simulink model "SF021A_HwAgTrajGenn"  (R2013b)
settings: Solver=FixedStepDiscrete  SolverMode=SingleTasking  StartTime=0.0  StopTime=1  FixedStep=0.002  RelTol=1e-3
undefined symbols (not defined in the file): ARCHGLBPRM_2MILLISEC_SEC_F32, HwAgTrajCmdSt1, HwAgTrajGennAgMax, HwAgTrajGennAMax, HwAgTrajGennVelMax, MINATAR_HWDEGPERSECPERSEC_F32, MINVELTAR_HWDEGPERSEC_F32, SYSGLBPRM_HWAGHILIM_HWDEG_F32, SYSGLBPRM_HWAGLOLIM_HWDEG_F32
libraries: simulink x13, NexteerUtilities x5
(part 2 of 2)

== system SF021A_HwAgTrajGenn/HwAgTrajGenn/HwAgTrajGennPer1/Generate Signals/Case 1/If Action Subsystem1 ==
  Cmd_St : Inport
  Ti_St : Inport  Port=2
  HwPosn_Offs : Inport  Port=3
  Action Port : ActionPort  ActionType=else
  CopyRight2 : Subsystem  Description=|  mask(Copyright Information){none=on}
      | Copyright info block.                                               
      |                                                                     
      | Place copyright information at the top of every subsystem in design.
      mask prompts: none "No parameters"
      mask help: Place copyright information at the top of every subsystem in design.
      mask Display:
      | NxtrConf = 'Nexteer Confidential';
      | 
      | sys = bdroot; %handle for the current model ("system")
      | first = get_param(sys,'Created');
      | if(isempty(first))
      |     first = datestr(now,'yyyy');
      | else
      |     first = first(end-3:end);  %year is last four digits
      | end
      | 
      | last = get_param(sys,'LastModifiedDate');
      | if isempty(last)
      |     last = datestr(now,'yyyy');
      | else
      |     last = last(end-3:end);
      | end
      | 
      | if strcmp(first,last)
      |     fprintf('%s -- Copyright %s Nexteer',NxtrConf,first)
      | else
      |     fprintf('%s -- %s%s- %s Nexteer',NxtrConf,char(169),first,last)
      | end
  Cmd_St_notDone : Outport
  Ti_St_notDone : Outport  Port=2
  HwPosn_Offs_notDone : Outport  Port=3
  wires:
  HwPosn_Offs/1 -> HwPosn_Offs_notDone/1
  Ti_St/1 -> Ti_St_notDone/1
  Cmd_St/1 -> Cmd_St_notDone/1

== system SF021A_HwAgTrajGenn/HwAgTrajGenn/HwAgTrajGennPer1/Generate Signals/Case 2/CopyRight2 ==

== system SF021A_HwAgTrajGenn/HwAgTrajGenn/HwAgTrajGennPer1/Generate Signals/Case 2/If Action Subsystem ==
  Cmd_St : Inport
  Ti_St : Inport  Port=2
  HwPosn_Offs : Inport  Port=3
  Action Port : ActionPort  ActionType=then
  CopyRight2 : Subsystem  Description=|  mask(Copyright Information){none=on}
      | Copyright info block.                                               
      |                                                                     
      | Place copyright information at the top of every subsystem in design.
      mask prompts: none "No parameters"
      mask help: Place copyright information at the top of every subsystem in design.
      mask Display:
      | NxtrConf = 'Nexteer Confidential';
      | 
      | sys = bdroot; %handle for the current model ("system")
      | first = get_param(sys,'Created');
      | if(isempty(first))
      |     first = datestr(now,'yyyy');
      | else
      |     first = first(end-3:end);  %year is last four digits
      | end
      | 
      | last = get_param(sys,'LastModifiedDate');
      | if isempty(last)
      |     last = datestr(now,'yyyy');
      | else
      |     last = last(end-3:end);
      | end
      | 
      | if strcmp(first,last)
      |     fprintf('%s -- Copyright %s Nexteer',NxtrConf,first)
      | else
      |     fprintf('%s -- %s%s- %s Nexteer',NxtrConf,char(169),first,last)
      | end
  Cmd_St_Done : Outport
  Ti_St_Done : Outport  Port=2
  HwPosn_Offs_Done : Outport  Port=3
  wires:
  HwPosn_Offs/1 -> HwPosn_Offs_Done/1
  Ti_St/1 -> Ti_St_Done/1
  Cmd_St/1 -> Cmd_St_Done/1

== system SF021A_HwAgTrajGenn/HwAgTrajGenn/HwAgTrajGennPer1/Generate Signals/Case 2/If Action Subsystem1 ==
  Cmd_St : Inport
  Ti_St : Inport  Port=2
  HwPosn_Offs : Inport  Port=3
  Action Port : ActionPort  ActionType=else
  CopyRight2 : Subsystem  Description=|  mask(Copyright Information){none=on}
      | Copyright info block.                                               
      |                                                                     
      | Place copyright information at the top of every subsystem in design.
      mask prompts: none "No parameters"
      mask help: Place copyright information at the top of every subsystem in design.
      mask Display:
      | NxtrConf = 'Nexteer Confidential';
      | 
      | sys = bdroot; %handle for the current model ("system")
      | first = get_param(sys,'Created');
      | if(isempty(first))
      |     first = datestr(now,'yyyy');
      | else
      |     first = first(end-3:end);  %year is last four digits
      | end
      | 
      | last = get_param(sys,'LastModifiedDate');
      | if isempty(last)
      |     last = datestr(now,'yyyy');
      | else
      |     last = last(end-3:end);
      | end
      | 
      | if strcmp(first,last)
      |     fprintf('%s -- Copyright %s Nexteer',NxtrConf,first)
      | else
      |     fprintf('%s -- %s%s- %s Nexteer',NxtrConf,char(169),first,last)
      | end
  Cmd_St_notDone : Outport
  Ti_St_notDone : Outport  Port=2
  HwPosn_Offs_notDone : Outport  Port=3
  wires:
  Cmd_St/1 -> Cmd_St_notDone/1
  Ti_St/1 -> Ti_St_notDone/1
  HwPosn_Offs/1 -> HwPosn_Offs_notDone/1

== system SF021A_HwAgTrajGenn/HwAgTrajGenn/HwAgTrajGennPer1/Generate Signals/Case 3/CopyRight2 ==

== system SF021A_HwAgTrajGenn/HwAgTrajGenn/HwAgTrajGennPer1/Generate Signals/Case 3/If Action Subsystem ==
  Cmd_St : Inport
  Ti_St : Inport  Port=2
  HwPosn_Offs : Inport  Port=3
  Action Port : ActionPort  ActionType=then
  CopyRight2 : Subsystem  Description=|  mask(Copyright Information){none=on}
      | Copyright info block.                                               
      |                                                                     
      | Place copyright information at the top of every subsystem in design.
      mask prompts: none "No parameters"
      mask help: Place copyright information at the top of every subsystem in design.
      mask Display:
      | NxtrConf = 'Nexteer Confidential';
      | 
      | sys = bdroot; %handle for the current model ("system")
      | first = get_param(sys,'Created');
      | if(isempty(first))
      |     first = datestr(now,'yyyy');
      | else
      |     first = first(end-3:end);  %year is last four digits
      | end
      | 
      | last = get_param(sys,'LastModifiedDate');
      | if isempty(last)
      |     last = datestr(now,'yyyy');
      | else
      |     last = last(end-3:end);
      | end
      | 
      | if strcmp(first,last)
      |     fprintf('%s -- Copyright %s Nexteer',NxtrConf,first)
      | else
      |     fprintf('%s -- %s%s- %s Nexteer',NxtrConf,char(169),first,last)
      | end
  Cmd_St_Done : Outport
  Ti_St_Done : Outport  Port=2
  HwPosn_Offs_Done : Outport  Port=3
  wires:
  HwPosn_Offs/1 -> HwPosn_Offs_Done/1
  Ti_St/1 -> Ti_St_Done/1
  Cmd_St/1 -> Cmd_St_Done/1

== system SF021A_HwAgTrajGenn/HwAgTrajGenn/HwAgTrajGennPer1/Generate Signals/Case 3/If Action Subsystem1 ==
  Cmd_St : Inport
  Ti_St : Inport  Port=2
  HwPosn_Offs : Inport  Port=3
  Action Port : ActionPort  ActionType=else
  CopyRight2 : Subsystem  Description=|  mask(Copyright Information){none=on}
      | Copyright info block.                                               
      |                                                                     
      | Place copyright information at the top of every subsystem in design.
      mask prompts: none "No parameters"
      mask help: Place copyright information at the top of every subsystem in design.
      mask Display:
      | NxtrConf = 'Nexteer Confidential';
      | 
      | sys = bdroot; %handle for the current model ("system")
      | first = get_param(sys,'Created');
      | if(isempty(first))
      |     first = datestr(now,'yyyy');
      | else
      |     first = first(end-3:end);  %year is last four digits
      | end
      | 
      | last = get_param(sys,'LastModifiedDate');
      | if isempty(last)
      |     last = datestr(now,'yyyy');
      | else
      |     last = last(end-3:end);
      | end
      | 
      | if strcmp(first,last)
      |     fprintf('%s -- Copyright %s Nexteer',NxtrConf,first)
      | else
      |     fprintf('%s -- %s%s- %s Nexteer',NxtrConf,char(169),first,last)
      | end
  Cmd_St_notDone : Outport
  Ti_St_notDone : Outport  Port=2
  HwPosn_Offs_notDone : Outport  Port=3
  wires:
  Cmd_St/1 -> Cmd_St_notDone/1
  Ti_St/1 -> Ti_St_notDone/1
  HwPosn_Offs/1 -> HwPosn_Offs_notDone/1

== system SF021A_HwAgTrajGenn/HwAgTrajGenn/HwAgTrajGennPer1/Generate Signals/Case 4/CopyRight2 ==

== system SF021A_HwAgTrajGenn/HwAgTrajGenn/HwAgTrajGennPer1/Initialize Variables/If Action Subsystem/CopyRight2 ==

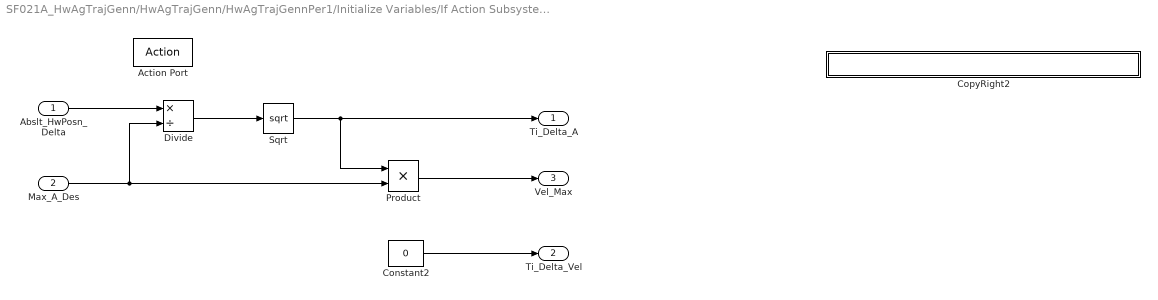
== system SF021A_HwAgTrajGenn/HwAgTrajGenn/HwAgTrajGennPer1/Initialize Variables/If Action Subsystem/|HwPosn_Delta|//2 < HwPosn_Delta_A_Des ==
  Abslt_HwPosn_Delta : Inport
  "Max_A_Des " : Inport  Port=2
  Action Port : ActionPort  ActionType=then
  Constant2 : Constant  Value=0  OutDataTypeStr=single
  CopyRight2 : Subsystem  Description=|  mask(Copyright Information){none=on}
      | Copyright info block.                                               
      |                                                                     
      | Place copyright information at the top of every subsystem in design.
      mask prompts: none "No parameters"
      mask help: Place copyright information at the top of every subsystem in design.
      mask Display:
      | NxtrConf = 'Nexteer Confidential';
      | 
      | sys = bdroot; %handle for the current model ("system")
      | first = get_param(sys,'Created');
      | if(isempty(first))
      |     first = datestr(now,'yyyy');
      | else
      |     first = first(end-3:end);  %year is last four digits
      | end
      | 
      | last = get_param(sys,'LastModifiedDate');
      | if isempty(last)
      |     last = datestr(now,'yyyy');
      | else
      |     last = last(end-3:end);
      | end
      | 
      | if strcmp(first,last)
      |     fprintf('%s -- Copyright %s Nexteer',NxtrConf,first)
      | else
      |     fprintf('%s -- %s%s- %s Nexteer',NxtrConf,char(169),first,last)
      | end
  Divide : Product  Inputs=*/
  Product : Product
  Sqrt : Sqrt  SaturateOnIntegerOverflow=on
  Ti_Delta_A : Outport
  Ti_Delta_Vel : Outport  Port=2
  Vel_Max : Outport  Port=3
  wires:
  Abslt_HwPosn_Delta/1 -> Divide/1
  "Max_A_Des "/1 -> Divide/2, Product/2
  Divide/1 -> Sqrt/1
  Sqrt/1 -> Ti_Delta_A/1, Product/1
  Product/1 -> Vel_Max/1
  Constant2/1 -> Ti_Delta_Vel/1

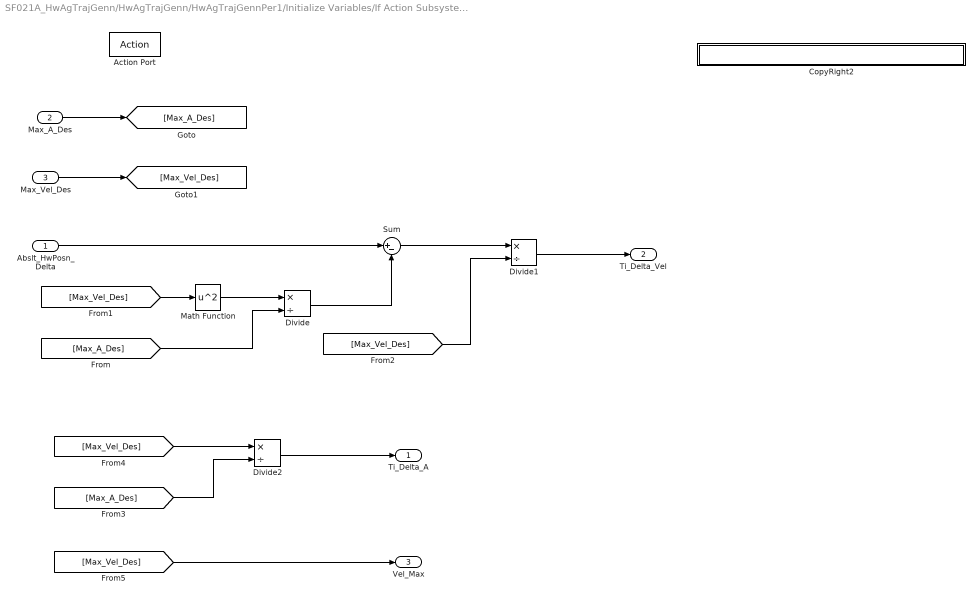
== system SF021A_HwAgTrajGenn/HwAgTrajGenn/HwAgTrajGennPer1/Initialize Variables/If Action Subsystem/|HwPosn_Delta|//2 >= HwPosn_Delta_A_Des ==
  Abslt_HwPosn_Delta : Inport
  Max_A_Des : Inport  Port=2
  Max_Vel_Des : Inport  Port=3
  Action Port : ActionPort  ActionType=else
  CopyRight2 : Subsystem  Description=|  mask(Copyright Information){none=on}
      | Copyright info block.                                               
      |                                                                     
      | Place copyright information at the top of every subsystem in design.
      mask prompts: none "No parameters"
      mask help: Place copyright information at the top of every subsystem in design.
      mask Display:
      | NxtrConf = 'Nexteer Confidential';
      | 
      | sys = bdroot; %handle for the current model ("system")
      | first = get_param(sys,'Created');
      | if(isempty(first))
      |     first = datestr(now,'yyyy');
      | else
      |     first = first(end-3:end);  %year is last four digits
      | end
      | 
      | last = get_param(sys,'LastModifiedDate');
      | if isempty(last)
      |     last = datestr(now,'yyyy');
      | else
      |     last = last(end-3:end);
      | end
      | 
      | if strcmp(first,last)
      |     fprintf('%s -- Copyright %s Nexteer',NxtrConf,first)
      | else
      |     fprintf('%s -- %s%s- %s Nexteer',NxtrConf,char(169),first,last)
      | end
  Divide : Product  Inputs=*/
  Divide1 : Product  Inputs=*/
  Divide2 : Product  Inputs=*/
  Math Function : Math  Operator=square  SaturateOnIntegerOverflow=on
  Sum : Sum  Inputs=|+-
  Ti_Delta_A : Outport
  Ti_Delta_Vel : Outport  Port=2
  Vel_Max : Outport  Port=3
  wires:
  Divide2/1 -> Ti_Delta_A/1
  [Max_Vel_Des] -> Vel_Max/1
  Divide1/1 -> Ti_Delta_Vel/1
  Max_A_Des/1 -> [Max_A_Des]
  Max_Vel_Des/1 -> [Max_Vel_Des]
  [Max_Vel_Des] -> Math Function/1
  Math Function/1 -> Divide/1
  [Max_A_Des] -> Divide/2
  Abslt_HwPosn_Delta/1 -> Sum/1
  Divide/1 -> Sum/2
  Sum/1 -> Divide1/1
  [Max_Vel_Des] -> Divide1/2
  [Max_Vel_Des] -> Divide2/1
  [Max_A_Des] -> Divide2/2

== system SF021A_HwAgTrajGenn/HwAgTrajGenn/HwAgTrajGennPer1/Generate Signals/Case 1/If Action Subsystem/CopyRight2 ==

== system SF021A_HwAgTrajGenn/HwAgTrajGenn/HwAgTrajGennPer1/Generate Signals/Case 1/If Action Subsystem1/CopyRight2 ==

== system SF021A_HwAgTrajGenn/HwAgTrajGenn/HwAgTrajGennPer1/Generate Signals/Case 2/If Action Subsystem/CopyRight2 ==

== system SF021A_HwAgTrajGenn/HwAgTrajGenn/HwAgTrajGennPer1/Generate Signals/Case 2/If Action Subsystem1/CopyRight2 ==

== system SF021A_HwAgTrajGenn/HwAgTrajGenn/HwAgTrajGennPer1/Generate Signals/Case 3/If Action Subsystem/CopyRight2 ==

== system SF021A_HwAgTrajGenn/HwAgTrajGenn/HwAgTrajGennPer1/Generate Signals/Case 3/If Action Subsystem1/CopyRight2 ==

== system SF021A_HwAgTrajGenn/HwAgTrajGenn/HwAgTrajGennPer1/Initialize Variables/If Action Subsystem/|HwPosn_Delta|//2 < HwPosn_Delta_A_Des/CopyRight2 ==

== system SF021A_HwAgTrajGenn/HwAgTrajGenn/HwAgTrajGennPer1/Initialize Variables/If Action Subsystem/|HwPosn_Delta|//2 >= HwPosn_Delta_A_Des/CopyRight2 ==
